simulink model "PI_continuo_graus"  (R2012b)
settings: Solver=ode45  StartTime=0.0  StopTime=100  RelTol=1e-3
settings Model: Creator=Walter  LastModifiedBy=Walter

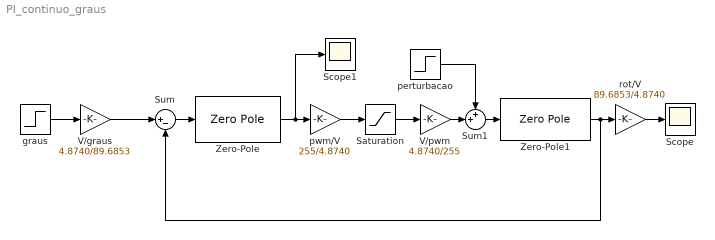
== system PI_continuo_graus ==
  Saturation : Saturate  UpperLimit=255  LowerLimit=-255
  Scope : Scope
  Scope1 : Scope
  Sum : Sum  Inputs=|+-
  Sum1 : Sum  Inputs=++|
  V/graus : Gain  Gain=4.8740/89.6853
  V/pwm : Gain  Gain=4.8740/255
  Zero-Pole : ZeroPole  Zeros=[-2.54]  Poles=[0]  Gain=[ 3.1368]
  Zero-Pole1 : ZeroPole  Zeros=[]  Poles=[0 -35.7143]  Gain=[110.4042]
  "graus " : Step  Time=0  After=1000  SampleTime=0
  perturbacao : Step  Time=0  After=0  SampleTime=0
  pwm/V : Gain  Gain=255/4.8740
  rot/V : Gain  Gain=89.6853/4.8740
  wires:
  "graus "/1 -> V/graus/1
  V/graus/1 -> Sum/1
  Sum/1 -> Zero-Pole/1
  Zero-Pole/1 -> Scope1/1, pwm/V/1
  pwm/V/1 -> Saturation/1
  Saturation/1 -> V/pwm/1
  V/pwm/1 -> Sum1/2
  perturbacao/1 -> Sum1/1
  Sum1/1 -> Zero-Pole1/1
  rot/V/1 -> Scope/1
  Zero-Pole1/1 -> Sum/2, rot/V/1
